simulink model "Simulink_non_linear_2controls_model"  (R2016a)
settings: Solver=ode45  SolverMode=SingleTasking  StartTime=0.0  StopTime=40  MaxStep=0.1  RelTol=1e-3
values from neighbouring files (symbols this model uses):
  M = csvread(filepath)    [txt2Map.m]
undefined symbols (not defined in the file or in its folder): g, m, MR, r, sigbuilder_block, TxBreak, TxCoulomb, TxVisc, TyBreak, TyCoulomb, TyVisc
settings Model: Creator=Roy  LastModifiedBy=Roy
settings DebuggingCC: SFUnexpectedBacktrackingDiag=error  SFNoUnconditionalDefaultTransitionDiag=error
settings GRTTargetCC: TargetLangStandard=C99 (ISO)  GeneratePreprocessorConditionals=Use local settings
settings ConfigComp: CovMetricSettings=dwe  CovHtmlReporting=off  CovSaveCumulativeToWorkspaceVar=off  CovSaveSingleToWorkspaceVar=off  CovExternalEMLEnable=on

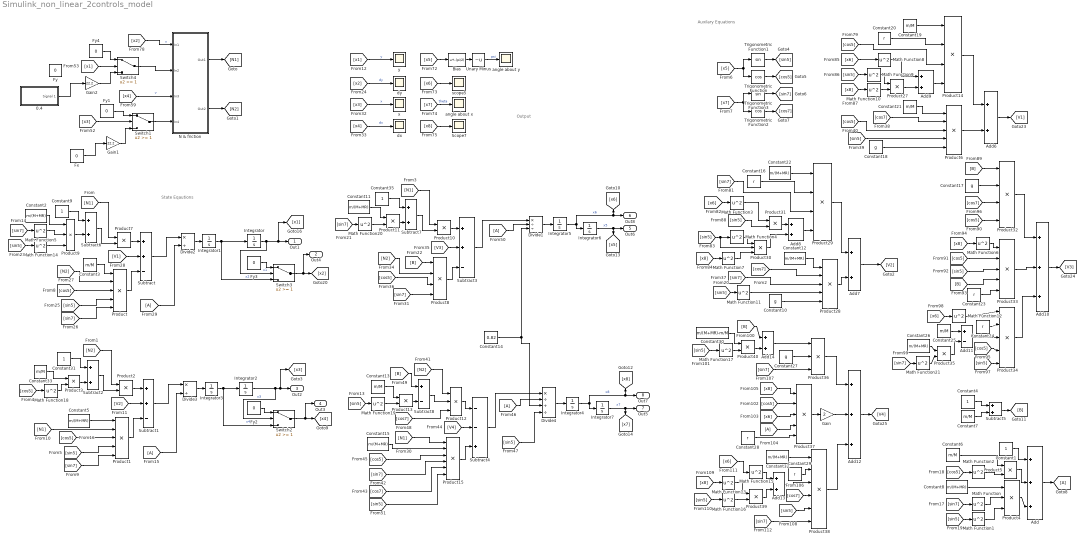
== system Simulink_non_linear_2controls_model ==
  note: Output
  note: State Eqautions
  note: Auxilary Equations
  0.4 : Subsystem  Tag=STV Subsys  LoadFcn=sigbuilder_block('load');  StartFcn=sigbuilder_block('start');  StopFcn=sigbuilder_block('stop');  ClipboardFcn=sigbuilder_block('clipboard');  mask(Sigbuilder block){}
      mask help: Simulink:masks:SigbuilderBlock_MD
      mask init:
      | if ~strcmp(get_param(bdroot(gcbh),'SimulationStatus'),'stopped') tuvar = sigbuilder_block('maskInit'); end
      settings: CopyFcn=sigbuilder_block('copy');  DeleteFcn=sigbuilder_block('delete');  ModelCloseFcn=sigbuilder_block('modelClose');  PreSaveFcn=sigbuilder_block('preSave');  PauseFcn=sigbuilder_block('pause');  ContinueFcn=sigbuilder_block('continue');  NameChangeFcn=sigbuilder_block('namechange');  OpenFcn=sigbuilder_block('open',[437.6 199.2 550.4 400 ]);  CloseFcn=sigbuilder_block('close');
      mask Display: plot(0, 0, 100, 100,[2, 2, 32, 32, 2], [68, 8, 8, 68, 68],[32, 2], [38, 38], [32, 19, 2],[53, 60, 44], [32, 17, 17, 2],[16, 16, 31, 31]);txt = getActiveGroup(gcbh);text(2, 100, txt,'verticalAlignment', 'top');
  Add : Sum  Inputs=+++
  Add10 : Sum  Inputs=+++
  Add11 : Sum  Inputs=+-
  Add12 : Sum  Inputs=+++
  Add{6..9,13..14} (6 alike) : Sum
  Bias : Bias  Bias=-(pi/2)
  Constant{1,4,9,31,35} (5 alike) : Constant
  Constant{10,17..18,27} (4 alike) : Constant  Value=g
  Constant{2,5,8,11..12,15,22,26,32} (9 alike) : Constant  Value=m/(M+MR)
  Constant{3,6..7,13,19,21,25,33} (8 alike) : Constant  Value=m/M
  Constant14 : Constant  Value=0.82
  Constant{16,20,23..24,28..29} (6 alike) : Constant  Value=r
  Constant30 : Constant  Value=m/(M+MR)-m/M
  Divide1 : Product  Inputs=*//
  Divide2 : Product  Inputs=*/
  Divide3 : Product  Inputs=*/
  Divide4 : Product  Inputs=*///
  Fx : Constant  Value=0
  Fy{,1..4} (5 alike) : Constant  Value=0
  Gain : Gain  Gain=2
  Gain1 : Gain  Gain=22.2
  Gain2 : Gain  Gain=22.2
  Integrator : Integrator  LimitOutput=on  UpperSaturationLimit=1  LowerSaturationLimit=0
  Integrator{1,3..5,7} (5 alike) : Integrator
  Integrator2 : Integrator  LimitOutput=on  UpperSaturationLimit=1  LowerSaturationLimit=0
  Integrator6 : Integrator  InitialCondition=pi/2
  Math Function{,1..21} (22 alike) : Math  Operator=square  SaturateOnIntegerOverflow=on
  N & friction : Subsystem
  Product{,1,6,28,33..34,37} (7 alike) : Product  Inputs=5
  Product{2..3,5,7,10..11,13,27,31,35,39..40} (12 alike) : Product
  Product{4,9,12,30,36} (5 alike) : Product  Inputs=3
  Product{8,14,29,32} (4 alike) : Product  Inputs=4
  Product15 : Product  Inputs=6
  Product38 : Product  Inputs=6
  Scope7 : Scope
  Subtract : Sum  Inputs=++-
  Subtract1 : Sum  Inputs=++-
  Subtract2 : Sum  Inputs=2
  Subtract3 : Sum  Inputs=++-
  Subtract4 : Sum  Inputs=--+
  Subtract5 : Sum
  Subtract6 : Sum  Inputs=2
  Subtract7 : Sum  Inputs=2
  Subtract8 : Sum  Inputs=+-
  Switch{1..4} (4 alike) : Switch  Threshold=1
  Trigonometric Function : Trigonometry  Operator=cos
  Trigonometric Function1 : Trigonometry
  Trigonometric Function2 : Trigonometry  Operator=cos
  Trigonometric Function3 : Trigonometry
  Unary Minus : UnaryMinus
  angle about x : Scope
  angle about y : Scope
  dx : Scope
  dy : Scope
  scope5 : Scope
  x : Scope
  y : Scope
  Out1 : Outport
  Out4 : Outport  Port=2
  Out2 : Outport  Port=3
  Out3 : Outport  Port=4
  Out6 : Outport  Port=5
  Out8 : Outport  Port=6
  Out5 : Outport  Port=7
  Out7 : Outport  Port=8
  wires:
  Constant3/1 -> Product/1
  Integrator1/1 -> Switch3/3, Integrator/1  "x2"
  [x5] -> Trigonometric Function/1, Trigonometric Function1/1
  [x7] -> Trigonometric Function3/1, Trigonometric Function2/1
  Trigonometric Function/1 -> [cos5]
  Trigonometric Function3/1 -> [sin7]
  Trigonometric Function2/1 -> [cos7]
  Trigonometric Function1/1 -> [sin5]
  [cos5] -> Product/3
  Constant8/1 -> Product4/1
  Subtract5/1 -> [B]
  Integrator6/1 -> [x5], Out6/1  "x5"
  Subtract3/1 -> Divide1/1
  Divide1/1 -> Integrator5/1
  [A] -> Divide1/2
  [x1] -> y/1  "y"
  [x2] -> dy/1  "dy"
  [x3] -> x/1  "x"
  [x4] -> dx/1  "dx"
  [x5] -> Bias/1
  [x8] -> Scope7/1
  [x7] -> angle about x/1  "theta"
  [x6] -> scope5/1
  Integrator5/1 -> [x6], Out8/1, Integrator6/1  "x6"
  [x2] -> N & friction/1(In1)  "v"
  [x4] -> N & friction/3(In3)  "v"
  N & friction/1(Out1) -> [N1]
  N & friction/2(Out2) -> [N2]
  Add/1 -> [A]
  [sin7] -> Math Function/1
  Math Function/1 -> Product4/2
  [sin5] -> Math Function1/1
  Math Function1/1 -> Product4/3
  [cos5] -> Math Function2/1
  Product4/1 -> Add/3
  Product5/1 -> Add/2
  Math Function2/1 -> Product5/2
  Constant6/1 -> Product5/1
  Constant1/1 -> Add/1
  Constant7/1 -> Subtract5/2
  Constant4/1 -> Subtract5/1
  Product28/1 -> Add7/2
  Product29/1 -> Add7/1
  Add7/1 -> [V2]
  Constant22/1 -> Product29/1
  Constant16/1 -> Product29/2
  [sin7] -> Product29/3
  [x6] -> Math Function3/1
  Product30/1 -> Add8/2
  Math Function4/1 -> Product30/1
  [x8] -> Math Function7/1
  Add8/1 -> Product29/4
  Constant10/1 -> Product28/5
  [sin5] -> Math Function11/1
  [sin7] -> Product28/3
  [cos7] -> Product28/2
  Constant12/1 -> Product28/1
  Constant21/1 -> Product6/1
  [cos7] -> Product6/2
  [cos5] -> Product6/3
  [sin5] -> Product6/4
  Constant18/1 -> Product6/5
  Add9/1 -> Product14/4
  Math Function10/1 -> Product27/2
  [x8] -> Math Function10/1
  Math Function9/1 -> Product27/1
  Product27/1 -> Add9/2
  [sin5] -> Math Function9/1
  Math Function8/1 -> Add9/1
  [x6] -> Math Function8/1
  [cos5] -> Product14/3
  Constant20/1 -> Product14/2
  Constant19/1 -> Product14/1
  Add6/1 -> [V1]
  Product14/1 -> Add6/1
  Product6/1 -> Add6/2
  Product31/1 -> Add8/1
  Math Function3/1 -> Product31/1
  [sin5] -> Product31/2
  [sin5] -> Product30/2, Math Function4/1
  Math Function7/1 -> Product30/3
  Math Function11/1 -> Product28/4
  [sin5] -> Product33/3
  [B] -> Product32/1
  Product32/1 -> Add10/1
  [cos5] -> Product33/2
  [x8] -> Math Function6/1
  Product33/1 -> Add10/2
  Product34/1 -> Add10/3
  Add10/1 -> [V3]
  Constant17/1 -> Product32/2
  [cos7] -> Product32/3
  [cos5] -> Product32/4
  Math Function6/1 -> Product33/1
  [B] -> Product33/4
  Constant23/1 -> Product33/5
  [sin5] -> Product34/5
  [cos5] -> Product34/4
  [x6] -> Math Function12/1
  Math Function12/1 -> Product34/1
  Constant24/1 -> Product34/2
  Add11/1 -> Product34/3
  Constant25/1 -> Add11/1
  Product35/1 -> Add11/2
  Constant26/1 -> Product35/1
  [sin5] -> Math Function16/1
  Product39/1 -> Add13/2
  Add13/1 -> Product38/3
  Constant29/1 -> Product38/2
  Constant32/1 -> Product38/1
  [cos7] -> Product38/4
  [sin5] -> Product38/5
  Constant28/1 -> Product37/5
  [A] -> Product37/4
  [x8] -> Product37/1
  [sin7] -> Product36/3
  Constant27/1 -> Product36/2
  Add12/1 -> [V4]
  Product38/1 -> Add12/3
  Product37/1 -> Gain/1
  [cos5] -> Product37/2
  Product36/1 -> Add12/1
  [x6] -> Product37/3
  [x6] -> Math Function15/1
  Math Function15/1 -> Add13/1
  [x8] -> Math Function13/1
  Math Function16/1 -> Product39/2
  Math Function13/1 -> Product39/1
  [sin7] -> Product38/6
  [B] -> Add14/1
  Constant30/1 -> Product40/1
  Product40/1 -> Add14/2
  Math Function17/1 -> Product40/2
  [sin5] -> Math Function17/1
  Add14/1 -> Product36/1
  Gain/1 -> Add12/2
  [N1] -> Product7/1
  Subtract6/1 -> Product7/2
  Math Function14/1 -> Product9/3
  [sin5] -> Math Function14/1
  Math Function5/1 -> Product9/2
  [sin7] -> Math Function5/1
  Constant2/1 -> Product9/1
  Product9/1 -> Subtract6/2
  Constant9/1 -> Subtract6/1
  Product7/1 -> Subtract/1
  Product/1 -> Subtract/3
  [sin5] -> Product/4
  [sin7] -> Product/5
  [N2] -> Product/2
  [V1] -> Subtract/2
  Divide2/1 -> Integrator1/1
  Subtract/1 -> Divide2/1
  [A] -> Divide2/2
  [A] -> Divide3/2
  Subtract1/1 -> Divide3/1
  Divide3/1 -> Integrator3/1
  [V2] -> Subtract1/2
  [N1] -> Product1/2
  [sin7] -> Product1/5
  [sin5] -> Product1/4
  Product1/1 -> Subtract1/3
  Product2/1 -> Subtract1/1
  Constant31/1 -> Subtract2/1
  Product3/1 -> Subtract2/2
  [cos5] -> Math Function18/1
  Subtract2/1 -> Product2/2
  [N2] -> Product2/1
  [cos5] -> Product1/3
  Integrator3/1 -> Switch2/3, Integrator2/1  "x4"
  Constant5/1 -> Product1/1
  Integrator2/1 -> Switch2/2, Out2/1, [x3]  "x3"
  Constant33/1 -> Product3/1
  Math Function18/1 -> Product3/2
  [N1] -> Product10/1
  Subtract7/1 -> Product10/2
  Constant35/1 -> Subtract7/1
  [sin7] -> Math Function20/1
  Constant11/1 -> Product11/1
  Math Function20/1 -> Product11/2
  Product10/1 -> Subtract3/1
  [N2] -> Product8/2
  Product11/1 -> Subtract7/2
  [B] -> Product8/1
  [cos5] -> Product8/3
  [sin7] -> Product8/4
  [V3] -> Subtract3/2
  Product8/1 -> Subtract3/3
  Product15/1 -> Subtract4/3
  [V4] -> Subtract4/2
  [sin7] -> Product15/4
  [cos5] -> Product15/3
  [N1] -> Product15/1
  Product13/1 -> Subtract8/2
  Constant15/1 -> Product15/2
  Product12/1 -> Subtract4/1
  Math Function19/1 -> Product13/2
  Constant13/1 -> Product13/1
  [sin5] -> Math Function19/1
  [B] -> Subtract8/1
  Subtract8/1 -> Product12/2
  [N2] -> Product12/1
  Constant14/1 -> Divide4/3, Divide1/3
  Integrator4/1 -> Integrator7/1, Out7/1, [x8]  "x8"
  [A] -> Divide4/2
  Divide4/1 -> Integrator4/1
  Subtract4/1 -> Divide4/1
  [sin5] -> Divide4/4
  [cos7] -> Product12/3
  [cos7] -> Product15/5
  [sin5] -> Product15/6
  Math Function21/1 -> Product35/2
  [sin7] -> Math Function21/1
  Integrator7/1 -> Out5/1, [x7]  "x7"
  Switch1/1 -> N & friction/4(In4)
  [x3] -> Switch1/2
  Fy1/1 -> Switch1/1
  Switch2/1 -> Out3/1, [x4]
  Fy2/1 -> Switch2/1
  Integrator/1 -> Switch3/2, [x1], Out1/1  "x1"
  Switch3/1 -> Out4/1, [x2]
  Fy3/1 -> Switch3/1
  Switch4/1 -> N & friction/2(In2)
  [x1] -> Switch4/2
  Fy4/1 -> Switch4/1
  Gain1/1 -> Switch1/3
  Gain2/1 -> Switch4/3
  Bias/1 -> Unary Minus/1
  Unary Minus/1 -> angle about y/1  "psi"
  0.4/1(Signal 1) -> Gain2/1
  Fx/1 -> Gain1/1

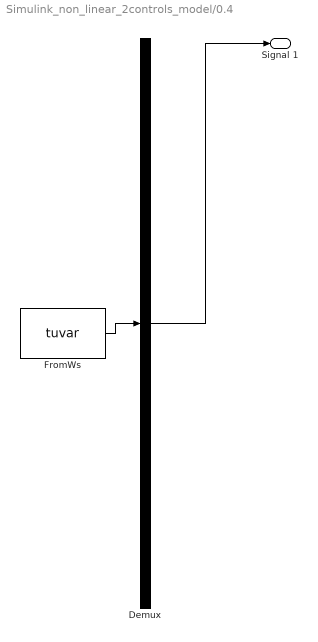
== system Simulink_non_linear_2controls_model/0.4 ==
  Demux : Demux  Tag=STV Demux  Outputs=1
  FromWs : FromWorkspace  Tag=STV FromWs  VariableName=tuvar  SampleTime=0
      SigBuilderData=|
      | common.afterFinalStr = 'Extrapolate'
      | common.sampleTime = 0
      | dataSet.timeRange = [0 10]
      | dataSet.name = 'Group 1'
      | sbobj.Groups.Name = 'Group 1'
      | sbobj.Groups.Signals.Name = 'Signal 1'
      | sbobj.Groups.Signals.XData = [0 1 1 2 2 10]
      | sbobj.Groups.Signals.YData = [0 0 0.8 0.8 0 0]
  Signal 1 : Outport  Tag=STV Outport
  wires:
  FromWs/1 -> Demux/1
  Demux/1 -> Signal 1/1

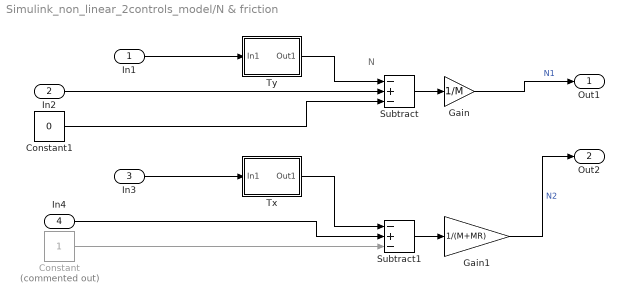
== system Simulink_non_linear_2controls_model/N & friction ==
  note: N
  In1 : Inport
  In2 : Inport  Port=2
  In3 : Inport  Port=3
  In4 : Inport  Port=4
  Constant : Constant  Commented=on
  Constant1 : Constant  Value=0
  Gain : Gain  Gain=1/M
  Gain1 : Gain  Gain=1/(M+MR)
  Subtract : Sum  Inputs=-+-
  Subtract1 : Sum  Inputs=-+-
  Tx : Subsystem
  Ty : Subsystem
  Out1 : Outport
  Out2 : Outport  Port=2
  wires:
  In1/1 -> Ty/1(In1)
  In3/1 -> Tx/1(In1)
  Subtract1/1 -> Gain1/1
  Gain1/1 -> Out2/1  "N2"
  In2/1 -> Subtract/2
  In4/1 -> Subtract1/2
  Subtract/1 -> Gain/1
  Tx/1(Out1) -> Subtract1/1
  Ty/1(Out1) -> Subtract/1
  Gain/1 -> Out1/1  "N1"
  Constant/1 -> Subtract1/3
  Constant1/1 -> Subtract/3

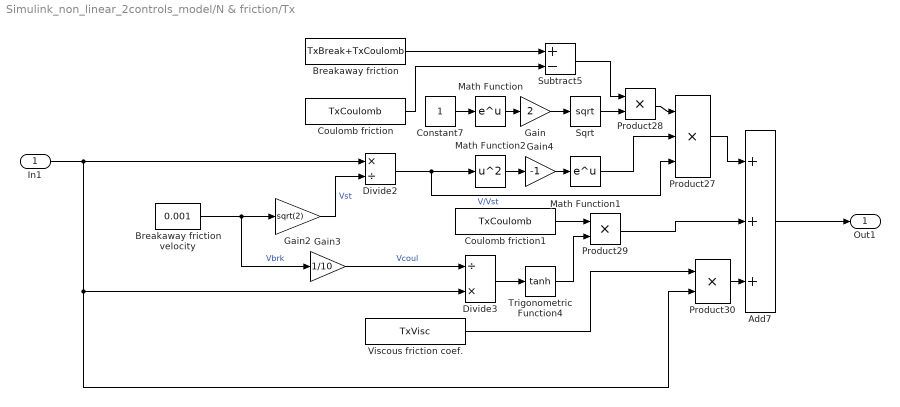
== system Simulink_non_linear_2controls_model/N & friction/Tx ==
  In1 : Inport
  Add7 : Sum  Inputs=+++
  Breakaway friction velocity : Constant  Value=0.001
  Breakaway friction : Constant  Value=TxBreak+TxCoulomb
  Constant7 : Constant
  Coulomb friction : Constant  Value=TxCoulomb
  Coulomb friction1 : Constant  Value=TxCoulomb
  Divide2 : Product  Inputs=*/
  Divide3 : Product  Inputs=/*
  Gain : Gain  Gain=2
  Gain2 : Gain  Gain=sqrt(2)
  Gain3 : Gain  Gain=1/10
  Gain4 : Gain  Gain=-1
  Math Function : Math  SaturateOnIntegerOverflow=on
  Math Function1 : Math  SaturateOnIntegerOverflow=on
  Math Function2 : Math  Operator=square  SaturateOnIntegerOverflow=on
  Product27 : Product  Inputs=3
  Product28 : Product
  Product29 : Product
  Product30 : Product
  Sqrt : Sqrt  SaturateOnIntegerOverflow=on
  Subtract5 : Sum  Inputs=+-
  Trigonometric Function4 : Trigonometry  Operator=tanh
  Viscous friction coef. : Constant  Value=TxVisc
  Out1 : Outport
  wires:
  Add7/1 -> Out1/1
  Divide2/1 -> Product27/3, Math Function2/1  "V/Vst"
  Product30/1 -> Add7/3
  Sqrt/1 -> Product28/2
  Product29/1 -> Add7/2
  Coulomb friction/1 -> Subtract5/2
  Subtract5/1 -> Product28/1
  Gain/1 -> Sqrt/1
  Product28/1 -> Product27/1
  Viscous friction coef./1 -> Product30/1
  Trigonometric Function4/1 -> Product29/2
  Breakaway friction/1 -> Subtract5/1
  Divide3/1 -> Trigonometric Function4/1
  Math Function/1 -> Gain/1
  Gain4/1 -> Math Function1/1
  Product27/1 -> Add7/1
  Breakaway friction velocity/1 -> Gain3/1, Gain2/1  "Vbrk"
  Math Function1/1 -> Product27/2
  Math Function2/1 -> Gain4/1
  Coulomb friction1/1 -> Product29/1
  Gain2/1 -> Divide2/2  "Vst"
  Constant7/1 -> Math Function/1
  In1/1 -> Divide3/2, Product30/2, Divide2/1
  Gain3/1 -> Divide3/1  "Vcoul"

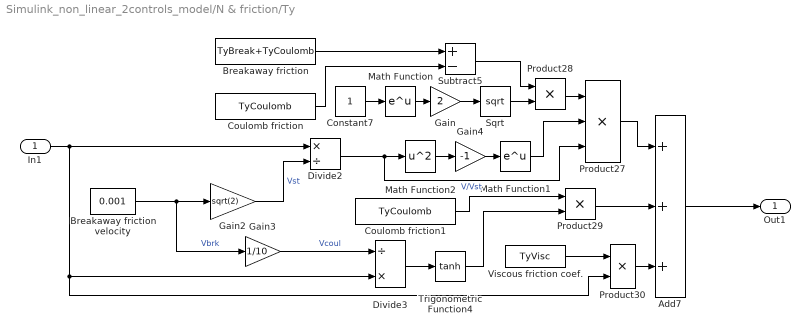
== system Simulink_non_linear_2controls_model/N & friction/Ty ==
  In1 : Inport
  Add7 : Sum  Inputs=+++
  Breakaway friction velocity : Constant  Value=0.001
  Breakaway friction : Constant  Value=TyBreak+TyCoulomb
  Constant7 : Constant
  Coulomb friction : Constant  Value=TyCoulomb
  Coulomb friction1 : Constant  Value=TyCoulomb
  Divide2 : Product  Inputs=*/
  Divide3 : Product  Inputs=/*
  Gain : Gain  Gain=2
  Gain2 : Gain  Gain=sqrt(2)
  Gain3 : Gain  Gain=1/10
  Gain4 : Gain  Gain=-1
  Math Function : Math  SaturateOnIntegerOverflow=on
  Math Function1 : Math  SaturateOnIntegerOverflow=on
  Math Function2 : Math  Operator=square  SaturateOnIntegerOverflow=on
  Product27 : Product  Inputs=3
  Product28 : Product
  Product29 : Product
  Product30 : Product
  Sqrt : Sqrt  SaturateOnIntegerOverflow=on
  Subtract5 : Sum  Inputs=+-
  Trigonometric Function4 : Trigonometry  Operator=tanh
  Viscous friction coef. : Constant  Value=TyVisc
  Out1 : Outport
  wires:
  Gain3/1 -> Divide3/1  "Vcoul"
  In1/1 -> Divide2/1, Product30/2, Divide3/2
  Constant7/1 -> Math Function/1
  Gain2/1 -> Divide2/2  "Vst"
  Coulomb friction1/1 -> Product29/1
  Math Function2/1 -> Gain4/1
  Math Function1/1 -> Product27/2
  Breakaway friction velocity/1 -> Gain2/1, Gain3/1  "Vbrk"
  Product27/1 -> Add7/1
  Gain4/1 -> Math Function1/1
  Math Function/1 -> Gain/1
  Divide3/1 -> Trigonometric Function4/1
  Breakaway friction/1 -> Subtract5/1
  Trigonometric Function4/1 -> Product29/2
  Viscous friction coef./1 -> Product30/1
  Product28/1 -> Product27/1
  Gain/1 -> Sqrt/1
  Subtract5/1 -> Product28/1
  Coulomb friction/1 -> Subtract5/2
  Product29/1 -> Add7/2
  Sqrt/1 -> Product28/2
  Product30/1 -> Add7/3
  Divide2/1 -> Math Function2/1, Product27/3  "V/Vst"
  Add7/1 -> Out1/1
